simulink model "sihPerceptionTest"  (R2026a)
settings: Solver=VariableStepAuto
settings Model: Creator=ROSHAN KUMAR C  LastModifiedBy=ROSHAN KUMAR C

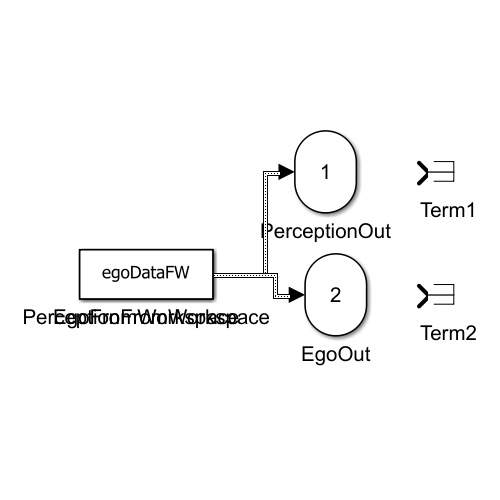
[thumbnail: Simulink's stored preview of the top-level diagram]
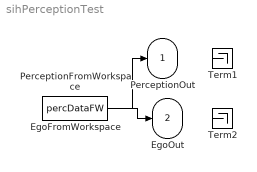
== system sihPerceptionTest ==
  EgoFromWorkspace : FromWorkspace  VariableName=egoDataFW  OutDataTypeStr=Bus: SihEgoBus  OutputAfterFinalValue=Holding final value
  PerceptionFromWorkspace : FromWorkspace  VariableName=percDataFW  OutDataTypeStr=Bus: SihPerceptionBus  Interpolate=off  OutputAfterFinalValue=Holding final value
  Term1 : Terminator
  Term2 : Terminator
  PerceptionOut : Outport
  EgoOut : Outport  Port=2
  wires:
  PerceptionFromWorkspace/1 -> PerceptionOut/1
  EgoFromWorkspace/1 -> EgoOut/1
